simulink model "FXP_AFMss_obshas_uk"  (R2016b)
settings: Solver=ode4  StartTime=0.0  StopTime=trun  FixedStep=Ts  RelTol=1e-5  EnableMultiTasking=on
PreLoadFcn:
  | VSS_CONTROL_MODE=1;
  | VSS_LINEAR_CONTROL=Simulink.Variant('VSS_CONTROL_MODE==1');
  | VSS_MPC_CONTROL=Simulink.Variant('VSS_CONTROL_MODE == 2');
  | 
  | 
  | VSS_STATE_DIRECT=Simulink.Variant('VSS_STATE_MODE==1');
  | VSS_STATE_OBS=Simulink.Variant('VSS_STATE_MODE==2');
  | VSS_STATE_DIST_OBS=Simulink.Variant('VSS_STATE_MODE==3');
  | VSS_STATE_MODE=1;
undefined symbols (not defined in the file): C_ydist, Ident_obs, PLANT, r, rp, sim_struct, Ts, w, wp, x0
libraries: cstblocks x2
settings Model: Creator=arnold  LastModifiedBy=arnold
settings DataIOCC: SaveFormat=Array  SaveOutput=off  SaveState=on  InspectSignalLogs=on  TimeSaveName=tout_ptos
settings OptimizationCC: LifeSpan=inf
settings DebuggingCC: SolverPrmCheckMsg=warning  SFUnexpectedBacktrackingDiag=warning  SFNoUnconditionalDefaultTransitionDiag=warning  SFExecutionAtInitializationDiag=none
settings HardwareCC: ProdBitPerPointer=32  ProdBitPerSizeT=32  ProdBitPerPtrDiffT=32  ProdLargestAtomicFloat=None  ProdIntDivRoundTo=Undefined  ProdEndianess=Unspecified  ProdWordSize=32  ProdHWDeviceType=32-bit Generic
settings ModelReferenceCC: PropagateSignalLabelsOutOfModel=off
settings GRTTargetCC: TargetLangStandard=C89/C90 (ANSI)  GeneratePreprocessorConditionals=Disable all
settings ConfigComp: CovMetricSettings=dw  CovHtmlReporting=on  CovSaveCumulativeToWorkspaceVar=on  CovSaveSingleToWorkspaceVar=on  CovExternalEMLEnable=off  CovSFcnEnable=off

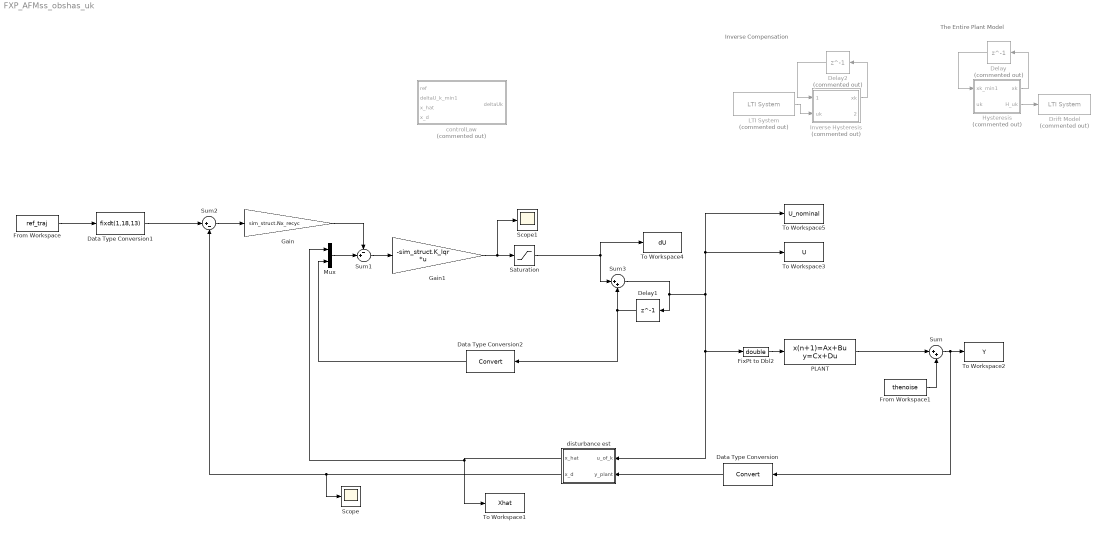
== system FXP_AFMss_obshas_uk ==
  note: Inverse Compensation
  note: The Entire Plant Model
  Data Type Conversion : DataTypeConversion
  Data Type Conversion1 : DataTypeConversion  OutDataTypeStr=fixdt(1,18,13)
  Data Type Conversion2 : DataTypeConversion
  Delay : Delay  Commented=on  DelayLength=1  InitialCondition=zeros(length(r),1)
  Delay1 : Delay  DelayLength=1  InitialCondition=0  SampleTime=Ts
  Delay2 : Delay  Commented=on  DelayLength=1  InitialCondition=zeros(length(rp),1)
  Drift Model : cstblocks/LTI System  Commented=on  sys=sim_struct.gdrift  IC=x0_full
  FixPt to Dbl2 : DataTypeConversion  OutDataTypeStr=double
  From Workspace : FromWorkspace  VariableName=ref_traj  SampleTime=Ts
  From Workspace1 : FromWorkspace  VariableName=thenoise  SampleTime=Ts
  Gain : Gain  Gain=sim_struct.Nx_recyc  OutDataTypeStr=fixdt(1,nw*2,32)
  Gain1 : Gain  Gain=-sim_struct.K_lqr  Multiplication=Matrix(K*u)  OutDataTypeStr=fixdt(1,nw,nf)
  Hysteresis : MATLAB Function  Commented=on  TreatAsAtomicUnit=on
  Inverse Hysteresis : MATLAB Function  Commented=on  TreatAsAtomicUnit=on
  LTI System : cstblocks/LTI System  Commented=on  sys=sim_struct.gdrift_inv  IC=[]
  Mux : Mux  Inputs=2
  PLANT : DiscreteStateSpace  A=PLANT.a  B=PLANT.b  C=PLANT.c  D=zeros(size(PLANT.c,1),1)  X0=x0  SampleTime=Ts
  Saturation : Saturate  UpperLimit=sim_struct.du_max  LowerLimit=-sim_struct.du_max
  Scope : Scope
  Scope1 : Scope
  Sum : Sum  Inputs=|++
  Sum1 : Sum  Inputs=-+|  OutDataTypeStr=fixdt(1,nw,nf)
  Sum2 : Sum  Inputs=|+-
  Sum3 : Sum  Inputs=|++
  To Workspace1 : ToWorkspace  VariableName=Xhat  SaveFormat=Timeseries  SampleTime=-1
      settings: Save2DSignal=2-D array (concatenate along first dimension)
  To Workspace2 : ToWorkspace  VariableName=Y  SaveFormat=Timeseries  SampleTime=-1
      settings: Save2DSignal=2-D array (concatenate along first dimension)
  To Workspace3 : ToWorkspace  VariableName=U  SaveFormat=Timeseries  SampleTime=-1
      settings: Save2DSignal=2-D array (concatenate along first dimension)
  To Workspace4 : ToWorkspace  VariableName=dU  SaveFormat=Timeseries  SampleTime=-1
      settings: Save2DSignal=2-D array (concatenate along first dimension)
  To Workspace5 : ToWorkspace  VariableName=U_nominal  SaveFormat=Timeseries  SampleTime=-1
      settings: Save2DSignal=2-D array (concatenate along first dimension)
  controlLaw : Subsystem  Commented=on
  disturbance est : Subsystem  VariantControl=VSS_STATE_DIST_OBS
  wires:
  Sum/1 -> Data Type Conversion/1, To Workspace2/1
  disturbance est/1(x_hat) -> Mux/1, To Workspace1/1
  From Workspace1/1 -> Sum/2
  PLANT/1 -> Sum/1
  Delay1/1 -> Data Type Conversion2/1, Sum3/2
  FixPt to Dbl2/1 -> PLANT/1
  Sum3/1 -> To Workspace3/1, To Workspace5/1, FixPt to Dbl2/1, disturbance est/1(u_of_k), Delay1/1
  Saturation/1 -> Sum3/1, To Workspace4/1
  From Workspace/1 -> Data Type Conversion1/1
  disturbance est/2(x_d) -> Sum2/2, Scope/1
  LTI System/1 -> Inverse Hysteresis/2(uk)
  Inverse Hysteresis/1(xk) -> Delay2/1
  Delay2/1 -> Inverse Hysteresis/1(xk_min1)
  Data Type Conversion1/1 -> Sum2/1
  Data Type Conversion/1 -> disturbance est/2(y_plant)
  Gain1/1 -> Scope1/1, Saturation/1
  Sum1/1 -> Gain1/1
  Mux/1 -> Sum1/2
  Gain/1 -> Sum1/1
  Data Type Conversion2/1 -> Mux/2
  Sum2/1 -> Gain/1
  Hysteresis/2(H_uk) -> Drift Model/1
  Hysteresis/1(xk) -> Delay/1
  Delay/1 -> Hysteresis/1(xk_min1)

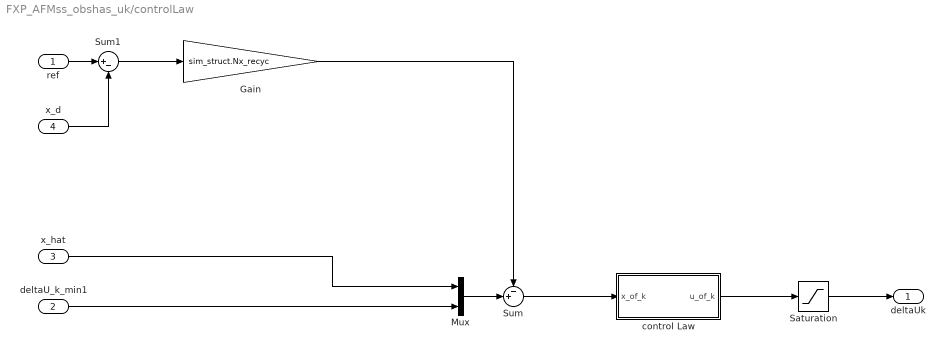
== system FXP_AFMss_obshas_uk/controlLaw ==
  ref : Inport
  deltaU_k_min1 : Inport  Port=2
  x_hat : Inport  Port=3
  x_d : Inport  Port=4
  Gain : Gain  Gain=sim_struct.Nx_recyc  OutDataTypeStr=fixdt(1,nw,nf)
  Mux : Mux  Inputs=2
  Saturation : Saturate  UpperLimit=sim_struct.du_max  LowerLimit=-sim_struct.du_max
  Sum : Sum  Inputs=-+|  OutDataTypeStr=fixdt(1,nw,nf)
  Sum1 : Sum  Inputs=|+-
  control Law : Subsystem  Variant=on  OverrideUsingVariant=VSS_LINEAR_CONTROL
  deltaUk : Outport
  wires:
  Saturation/1 -> deltaUk/1
  control Law/1(u_of_k) -> Saturation/1
  ref/1 -> Sum1/1
  Sum/1 -> control Law/1(x_of_k)
  x_hat/1 -> Mux/1
  deltaU_k_min1/1 -> Mux/2
  Mux/1 -> Sum/2
  Gain/1 -> Sum/1
  Sum1/1 -> Gain/1
  x_d/1 -> Sum1/2

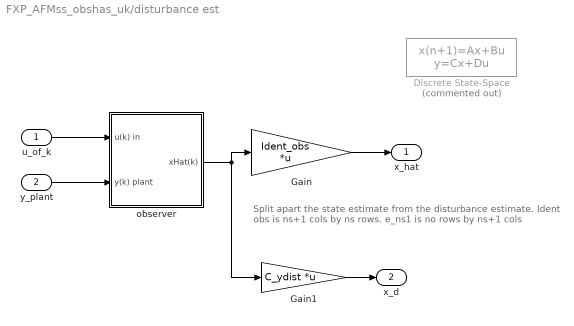
== system FXP_AFMss_obshas_uk/disturbance est ==
  note: Split apart the state estimate from the disturbance estimate.
      | Ident obs is ns+1 cols by ns rows. e_ns1 is no rows by ns+1 cols
  u_of_k : Inport
  y_plant : Inport  Port=2
  Discrete State-Space : DiscreteStateSpace  Commented=on  A=sim_struct.sys_obs.a  B=[sim_struct.sys_obs.b, sim_struct.L]  C=eye(length(sim_struct.sys_obs.b))  D=zeros(length(sim_struct.sys_obs.b), 2)  X0=sim_struct.x0_obs  SampleTime=Ts
  Gain : Gain  Gain=Ident_obs  Multiplication=Matrix(K*u)
  Gain1 : Gain  Gain=C_ydist  Multiplication=Matrix(K*u)
  observer : Subsystem
  x_hat : Outport
  x_d : Outport  Port=2
  wires:
  u_of_k/1 -> observer/1(u(k) in)
  observer/1(xHat(k)) -> Gain/1, Gain1/1
  y_plant/1 -> observer/2(y(k) plant)
  Gain/1 -> x_hat/1
  Gain1/1 -> x_d/1

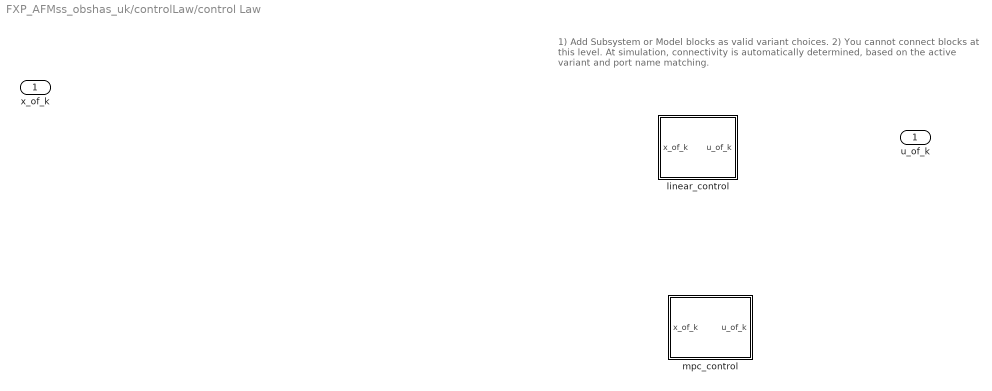
== system FXP_AFMss_obshas_uk/controlLaw/control Law ==
  note: 1) Add Subsystem or Model blocks as valid variant choices.
      | 2) You cannot connect blocks at this level. At simulation, connectivity is automatically
      | determined, based on the active variant and port name matching.
  x_of_k : Inport
  linear_control : Subsystem  VariantControl=VSS_LINEAR_CONTROL
  mpc_control : Subsystem  VariantControl=VSS_MPC_CONTROL
  u_of_k : Outport

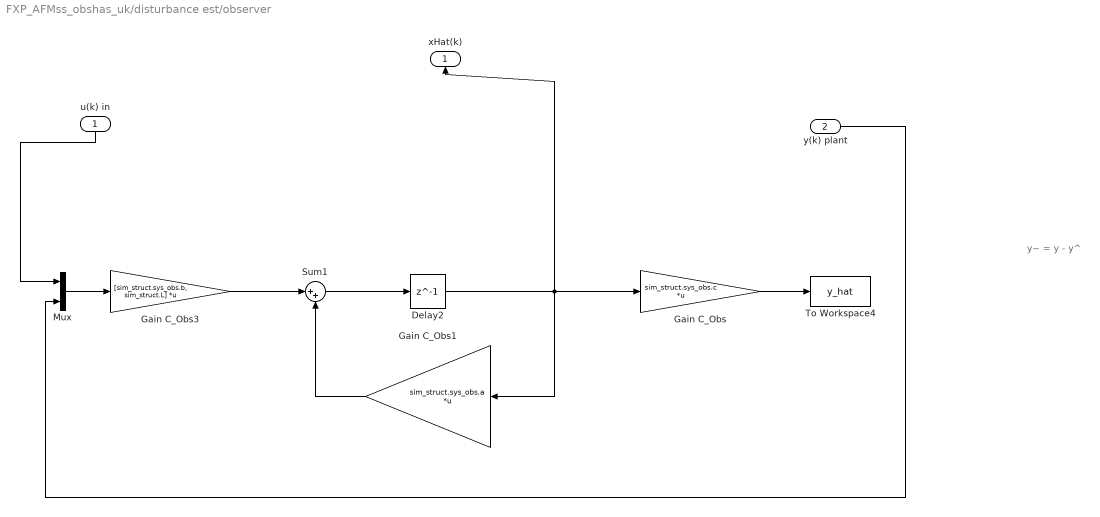
== system FXP_AFMss_obshas_uk/disturbance est/observer ==
  note: y~ = y - y^
  u(k) in : Inport
  y(k) plant : Inport  Port=2
  Delay2 : Delay  DelayLength=1  InitialCondition=sim_struct.x0_obs
  Gain C_Obs : Gain  Gain=sim_struct.sys_obs.c  Multiplication=Matrix(K*u)  OutDataTypeStr=fixdt(1,nw,nf)
  Gain C_Obs1 : Gain  Gain=sim_struct.sys_obs.a  Multiplication=Matrix(K*u)  OutDataTypeStr=fixdt(1,nw,nf)
  Gain C_Obs3 : Gain  Gain=[sim_struct.sys_obs.b, sim_struct.L]  Multiplication=Matrix(K*u)  OutDataTypeStr=fixdt(1,nw,nf)
  Mux : Mux  Inputs=2
  Sum1 : Sum  Inputs=|++  OutDataTypeStr=fixdt(1,nw,nf)
  To Workspace4 : ToWorkspace  VariableName=y_hat  SaveFormat=Timeseries  SampleTime=-1
      settings: Save2DSignal=2-D array (concatenate along first dimension)
  xHat(k) : Outport
  wires:
  Sum1/1 -> Delay2/1
  Gain C_Obs1/1 -> Sum1/2
  Mux/1 -> Gain C_Obs3/1
  y(k) plant/1 -> Mux/2
  Gain C_Obs/1 -> To Workspace4/1
  Delay2/1 -> xHat(k)/1, Gain C_Obs1/1, Gain C_Obs/1
  Gain C_Obs3/1 -> Sum1/1
  u(k) in/1 -> Mux/1

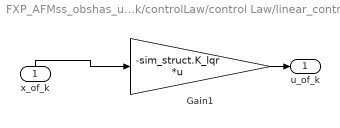
== system FXP_AFMss_obshas_uk/controlLaw/control Law/linear_control ==
  x_of_k : Inport
  Gain1 : Gain  Gain=-sim_struct.K_lqr  Multiplication=Matrix(K*u)  OutDataTypeStr=fixdt(1,nw,nf)
  u_of_k : Outport
  wires:
  x_of_k/1 -> Gain1/1
  Gain1/1 -> u_of_k/1

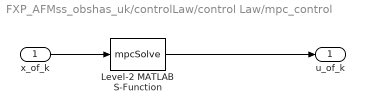
== system FXP_AFMss_obshas_uk/controlLaw/control Law/mpc_control ==
  x_of_k : Inport
  Level-2 MATLAB S-Function : M-S-Function  FunctionName=mpcSolve  Parameters=sim_struct.mpcProb
  u_of_k : Outport
  wires:
  x_of_k/1 -> Level-2 MATLAB S-Function/1
  Level-2 MATLAB S-Function/1 -> u_of_k/1

== matlab function FXP_AFMss_obshas_uk/Inverse Hysteresis ==
  data: xk output; xk_min1 input; uk input; H_inv_uk output; rp parameter; wp parameter
function [xk, H_inv_uk] = fcn(xk_min1, uk, rp, wp)
  % Implement simple IP hysteresis model.
  if length(rp) > 1
    xk = rp(:)*0;
    for j = 1:length(rp)
      xk(j) = max(uk - rp(j), min(uk+rp(j), xk_min1(j)));
    end
    
    H_inv_uk = wp'*xk(:);
  else
    xk = xk_min1;
    H_inv_uk = uk;
  end
end

== matlab function FXP_AFMss_obshas_uk/Hysteresis ==
  data: xk output; xk_min1 input; uk input; H_uk output; r parameter; w parameter
function [xk, H_uk] = fcn(xk_min1, uk, r, w)
  % Implement simple IP hysteresis model.
  if length(r) > 1
    xk = r(:)*0;
    for j = 1:length(r)
      xk(j) = max(uk - r(j), min(uk+r(j), xk_min1(j)));
    end
    
    H_uk = w'*xk(:);
  else
    xk = xk_min1;
    H_uk = uk;
  end
end
